simulink model "simu"  (R2018b)
settings: Solver=VariableStepAuto  StartTime=0.0  StopTime=10.0  RelTol=1e-3
values from neighbouring files (symbols this model uses):
  a0 = 1    [lab4.m]
  a1 = 1    [lab4.m]
  b = 8    [lab4.m]
  du = 0    [lab4.m]
  u0 = 8    [lab4.m]
  x0 = 2    [lab4.m]
settings Model: Creator=wojciechkonury  LastModifiedBy=wojciechkonury

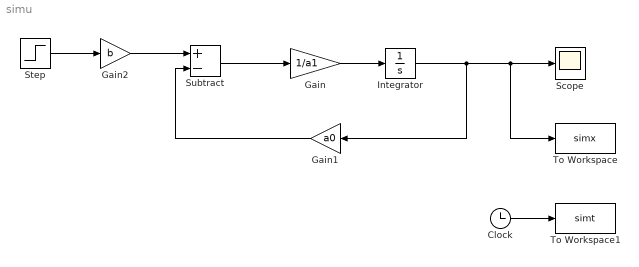
== system simu ==
  Clock : Clock
  Gain : Gain  Gain=1/a1
  Gain1 : Gain  Gain=a0
  Gain2 : Gain  Gain=b
  Integrator : Integrator  InitialCondition=x0
  Scope : Scope
  Step : Step  Before=u0  After=u0 + du  SampleTime=0
  Subtract : Sum  Inputs=+-
  To Workspace : ToWorkspace  VariableName=simx  SampleTime=-1
      settings: Save2DSignal=2-D array (concatenate along first dimension)
  To Workspace1 : ToWorkspace  VariableName=simt  SampleTime=-1
      settings: Save2DSignal=2-D array (concatenate along first dimension)
  wires:
  Gain/1 -> Integrator/1
  Gain1/1 -> Subtract/2
  Integrator/1 -> To Workspace/1, Scope/1, Gain1/1
  Subtract/1 -> Gain/1
  Gain2/1 -> Subtract/1
  Step/1 -> Gain2/1
  Clock/1 -> To Workspace1/1
